simulink model "plantaNeural"  (Simulink 7.4)
settings: Solver=ode45  StartTime=0.0  StopTime=10000  RelTol=1e-3
undefined symbols (not defined in the file or in its folder): now
libraries: neural x29, simulink_extras x2
settings Model: Creator=marco  LastModifiedBy=marco

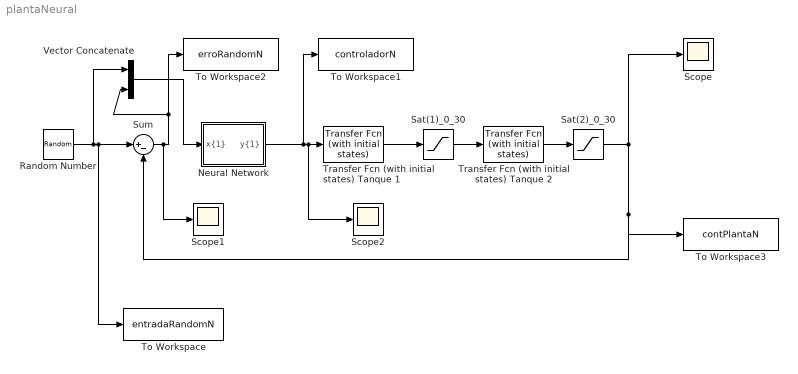
== system plantaNeural ==
  Neural Network : Subsystem
  Random Number : RandomNumber  Mean=15  Variance=15  Seed=round(now)  SampleTime=500
  Sat(1)_0_30 : Saturate  UpperLimit=30  LowerLimit=0  SampleTime=0.1  OutDataType=fixdt(1, 16)  OutScaling=2^0
  Sat(2)_0_30 : Saturate  UpperLimit=30  LowerLimit=0  SampleTime=0.1  OutDataType=fixdt(1, 16)  OutScaling=2^0
  Scope : Scope
  Scope1 : Scope
  Scope2 : Scope
      settings: YMin=4  YMax=5.5  SaveName=ScopeData2
  Sum : Sum  Inputs=|+-  OutDataType=fixdt(1, 16)  OutScaling=2^0  SampleTime=0.1
  To Workspace : ToWorkspace  VariableName=entradaRandomN  SampleTime=0.1  SaveFormat=Array
  To Workspace1 : ToWorkspace  VariableName=controladorN  SampleTime=0.1  SaveFormat=Array
  To Workspace2 : ToWorkspace  VariableName=erroRandomN  SampleTime=0.1  SaveFormat=Array
  To Workspace3 : ToWorkspace  VariableName=contPlantaN  SampleTime=0.1  SaveFormat=Array
  Transfer Fcn (with initial states) Tanque 1 : simulink_extras/Additional Linear/Transfer Fcn (with initial states)  SystemSampleTime=-1  N=[0.2964]  D="[1  0.0656]"  X0=0
  Transfer Fcn (with initial states) Tanque 2 : simulink_extras/Additional Linear/Transfer Fcn (with initial states)  SystemSampleTime=-1  N=[0.0656]  D="[1  0.0656]"  X0=0
  Vector Concatenate : Concatenate  Mode=Vector
  wires:
  Transfer Fcn (with initial states) Tanque 1/1 -> Sat(1)_0_30/1
  Sum/1 -> Scope1/1, To Workspace2/1, Vector Concatenate/2
  Transfer Fcn (with initial states) Tanque 2/1 -> Sat(2)_0_30/1
  Neural Network/1("y{1}") -> To Workspace1/1, Transfer Fcn (with initial states) Tanque 1/1, Scope2/1
  Random Number/1 -> To Workspace/1, Sum/1, Vector Concatenate/1
  Sat(1)_0_30/1 -> Transfer Fcn (with initial states) Tanque 2/1
  Sat(2)_0_30/1 -> Scope/1, Sum/2, To Workspace3/1
  Vector Concatenate/1 -> Neural Network/1("x{1}")

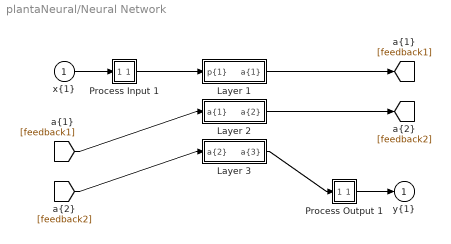
== system plantaNeural/Neural Network ==
  "x{1}" : Inport  PortDimensions=2  SampleTime=1
  Layer 1 : Subsystem
  Layer 2 : Subsystem
  Layer 3 : Subsystem
  Process Input 1 : Subsystem
  Process Output 1 : Subsystem
  "y{1}" : Outport  InitialOutput=0
  wires:
  "x{1}"/1 -> Process Input 1/1(x)
  Process Output 1/1(y) -> "y{1}"/1
  Process Input 1/1(p) -> Layer 1/1("p{1}")
  Layer 1/1("a{1}") -> [feedback1]
  [feedback1] -> Layer 2/1("a{1} ")
  Layer 2/1("a{2}") -> [feedback2]
  [feedback2] -> Layer 3/1("a{2} ")
  Layer 3/1("a{3}") -> Process Output 1/1(a)

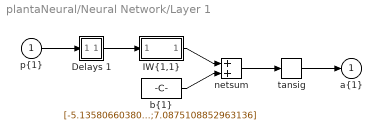
== system plantaNeural/Neural Network/Layer 1 ==
  "p{1}" : Inport  PortDimensions=2  SampleTime=1
  Delays 1 : Subsystem
      mask Display: disp('TDL')
  "IW{1,1}" : Subsystem
      mask Display: disp('weight')
  "b{1}" : Constant  Value=[-5.1358066038064774;-4.3696122158586421;-1.6705858835536853;-2.5464222267076702;-6.160408589801782;0.49822019697729519;-8.1445150751717037;5.2185710150424915;5.2648040348684608;7.0875108852963136]
      mask Display: disp('bias')
  netsum : Sum  Inputs=2  OutDataType=sfix(16)  OutScaling=2^0  SaturateOnIntegerOverflow=on  InputSameDT=on  OutDataTypeStr=Inherit: Same as first input
  tansig : neural/Transfer Functions/tansig  SystemSampleTime=-1
  "a{1}" : Outport  InitialOutput=[0;0;0;0;0;0;0;0;0;0]
  wires:
  "p{1}"/1 -> Delays 1/1("p{1}")
  Delays 1/1("pd{1,1}") -> "IW{1,1}"/1("pd{1,1}")
  "IW{1,1}"/1("iz{1,1}") -> netsum/1
  "b{1}"/1 -> netsum/2
  netsum/1 -> tansig/1
  tansig/1 -> "a{1}"/1

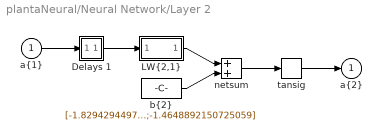
== system plantaNeural/Neural Network/Layer 2 ==
  "a{1} " : Inport  PortDimensions=10  SampleTime=1
  Delays 1 : Subsystem
      mask Display: disp('TDL')
  "LW{2,1}" : Subsystem
      mask Display: disp('weight')
  "b{2}" : Constant  Value=[-1.8294294497199188;2.7561117201367602;-1.1232541464035077;-1.6815661651128024;0.45024471298237856;0.059898257675119207;1.4208618932994941;-4.0307578032176012;0.90781113420925352;-1.4648892150725059]
      mask Display: disp('bias')
  netsum : Sum  Inputs=2  OutDataType=sfix(16)  OutScaling=2^0  SaturateOnIntegerOverflow=on  InputSameDT=on  OutDataTypeStr=Inherit: Same as first input
  tansig : neural/Transfer Functions/tansig  SystemSampleTime=-1
  "a{2}" : Outport  InitialOutput=[0;0;0;0;0;0;0;0;0;0]
  wires:
  "a{1} "/1 -> Delays 1/1("p{2}")
  Delays 1/1("pd{2,1}") -> "LW{2,1}"/1("ad{2,1}")
  "LW{2,1}"/1("lz{2,1}") -> netsum/1
  "b{2}"/1 -> netsum/2
  netsum/1 -> tansig/1
  tansig/1 -> "a{2}"/1

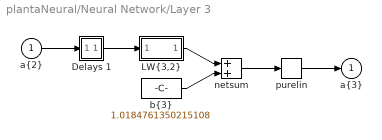
== system plantaNeural/Neural Network/Layer 3 ==
  "a{2} " : Inport  PortDimensions=10  SampleTime=1
  Delays 1 : Subsystem
      mask Display: disp('TDL')
  "LW{3,2}" : Subsystem
      mask Display: disp('weight')
  "b{3}" : Constant  Value=1.0184761350215108
      mask Display: disp('bias')
  netsum : Sum  Inputs=2  OutDataType=sfix(16)  OutScaling=2^0  SaturateOnIntegerOverflow=on  InputSameDT=on  OutDataTypeStr=Inherit: Same as first input
  purelin : neural/Transfer Functions/purelin  SystemSampleTime=-1
  "a{3}" : Outport  InitialOutput=0
  wires:
  "a{2} "/1 -> Delays 1/1("p{3}")
  Delays 1/1("pd{3,2}") -> "LW{3,2}"/1("ad{3,2}")
  "LW{3,2}"/1("lz{3,2}") -> netsum/1
  "b{3}"/1 -> netsum/2
  netsum/1 -> purelin/1
  purelin/1 -> "a{3}"/1

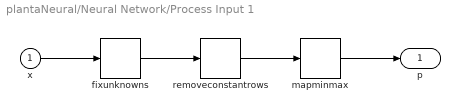
== system plantaNeural/Neural Network/Process Input 1 ==
  x : Inport  PortDimensions=2  SampleTime=1
  fixunknowns : neural/Processing Functions/fixunknowns  SystemSampleTime=-1  dummy=0
  mapminmax : neural/Processing Functions/mapminmax  SystemSampleTime=-1  xmin=[-5.46105933130547;1.67913647989072]  xmax=[23.6732986388822;29.4483698075216]  ymin=-1  ymax=1
  removeconstantrows : neural/Processing Functions/removeconstantrows  SystemSampleTime=-1  inputSize=2  keep=[1 2]
  p : Outport  PortDimensions=2  SampleTime=1
  wires:
  x/1 -> fixunknowns/1
  fixunknowns/1 -> removeconstantrows/1
  removeconstantrows/1 -> mapminmax/1
  mapminmax/1 -> p/1

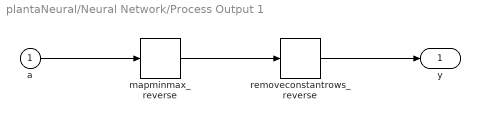
== system plantaNeural/Neural Network/Process Output 1 ==
  a : Inport  PortDimensions=1  SampleTime=1
  mapminmax_reverse : neural/Processing Functions/mapminmax_reverse  SystemSampleTime=-1  xmin=-15  xmax=15  ymin=-1  ymax=1
  removeconstantrows_reverse : neural/Processing Functions/removeconstantrows_reverse  SystemSampleTime=-1  inputSize=1  constants=zeros(0,1)  rearrange=1
  y : Outport  PortDimensions=1  SampleTime=1
  wires:
  a/1 -> mapminmax_reverse/1
  mapminmax_reverse/1 -> removeconstantrows_reverse/1
  removeconstantrows_reverse/1 -> y/1

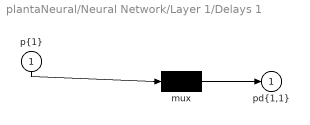
== system plantaNeural/Neural Network/Layer 1/Delays 1 ==
  "p{1}" : Inport  PortDimensions=2  SampleTime=1
  mux : Mux  Inputs=1
  "pd{1,1}" : Outport
  wires:
  "p{1}"/1 -> mux/1
  mux/1 -> "pd{1,1}"/1

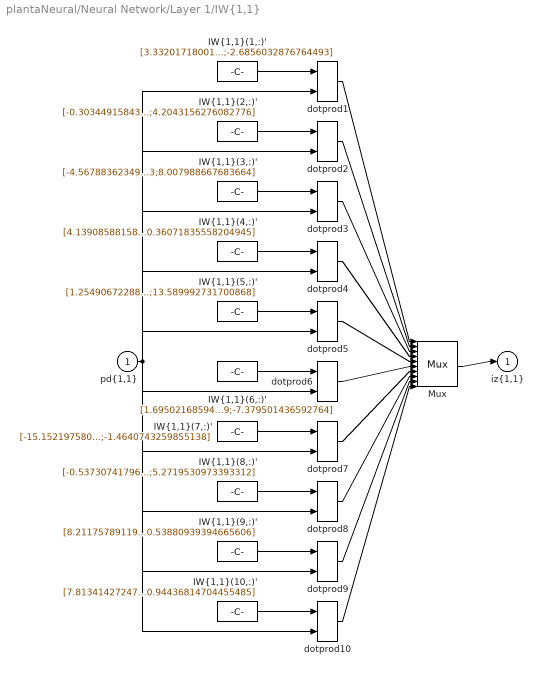
== system plantaNeural/Neural Network/Layer 1/IW{1,1} ==
  "pd{1,1}" : Inport  PortDimensions=2  SampleTime=1
  "IW{1,1}(1,:)'" : Constant  Value=[3.3320171800151712;-2.6856032876764493]
      mask Display: disp('weights')
  "IW{1,1}(10,:)'" : Constant  Value=[7.8134142724702738;0.94436814704455485]
      mask Display: disp('weights')
  "IW{1,1}(2,:)'" : Constant  Value=[-0.3034491584308816;4.2043156276082776]
      mask Display: disp('weights')
  "IW{1,1}(3,:)'" : Constant  Value=[-4.5678836234909763;8.007988667683664]
      mask Display: disp('weights')
  "IW{1,1}(4,:)'" : Constant  Value=[4.139085881580753;-0.36071835558204945]
      mask Display: disp('weights')
  "IW{1,1}(5,:)'" : Constant  Value=[1.2549067228851953;13.589992731700868]
      mask Display: disp('weights')
  "IW{1,1}(6,:)'" : Constant  Value=[1.6950216859409259;-7.379501436592764]
      mask Display: disp('weights')
  "IW{1,1}(7,:)'" : Constant  Value=[-15.152197580993475;-1.4640743259855138]
      mask Display: disp('weights')
  "IW{1,1}(8,:)'" : Constant  Value=[-0.53730741796460768;5.2719530973393312]
      mask Display: disp('weights')
  "IW{1,1}(9,:)'" : Constant  Value=[8.2117578911927342;-0.53880939394665606]
      mask Display: disp('weights')
  Mux : Mux  Inputs=10
  dotprod{1..10} (10 alike) : neural/Weight Functions/dotprod  SystemSampleTime=-1
  "iz{1,1}" : Outport
  wires:
  "IW{1,1}(1,:)'"/1 -> dotprod1/1
  "pd{1,1}"/1 -> dotprod1/2, dotprod2/2, dotprod3/2, dotprod4/2, dotprod5/2, dotprod6/2, dotprod7/2, dotprod8/2, dotprod9/2, dotprod10/2
  dotprod1/1 -> Mux/1
  "IW{1,1}(2,:)'"/1 -> dotprod2/1
  dotprod2/1 -> Mux/2
  "IW{1,1}(3,:)'"/1 -> dotprod3/1
  dotprod3/1 -> Mux/3
  "IW{1,1}(4,:)'"/1 -> dotprod4/1
  dotprod4/1 -> Mux/4
  "IW{1,1}(5,:)'"/1 -> dotprod5/1
  dotprod5/1 -> Mux/5
  "IW{1,1}(6,:)'"/1 -> dotprod6/1
  dotprod6/1 -> Mux/6
  "IW{1,1}(7,:)'"/1 -> dotprod7/1
  dotprod7/1 -> Mux/7
  "IW{1,1}(8,:)'"/1 -> dotprod8/1
  dotprod8/1 -> Mux/8
  "IW{1,1}(9,:)'"/1 -> dotprod9/1
  dotprod9/1 -> Mux/9
  "IW{1,1}(10,:)'"/1 -> dotprod10/1
  dotprod10/1 -> Mux/10
  Mux/1 -> "iz{1,1}"/1

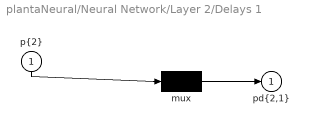
== system plantaNeural/Neural Network/Layer 2/Delays 1 ==
  "p{2}" : Inport  PortDimensions=10  SampleTime=1
  mux : Mux  Inputs=1
  "pd{2,1}" : Outport
  wires:
  "p{2}"/1 -> mux/1
  mux/1 -> "pd{2,1}"/1

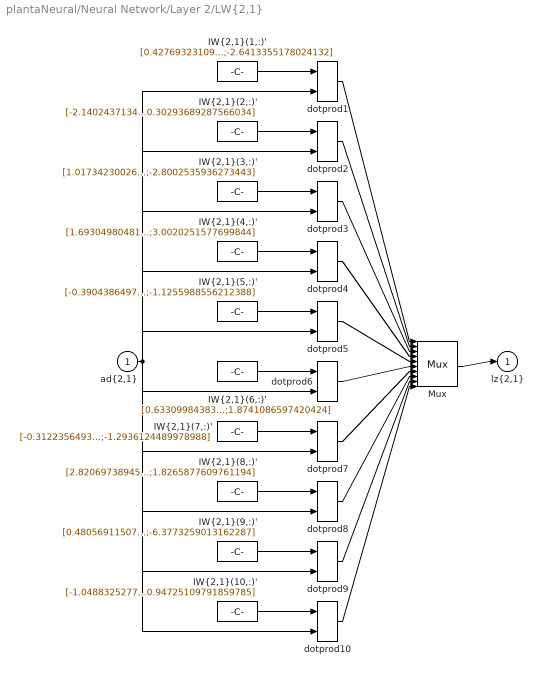
== system plantaNeural/Neural Network/Layer 2/LW{2,1} ==
  "ad{2,1}" : Inport  PortDimensions=10  SampleTime=1
  "IW{2,1}(1,:)'" : Constant  Value=[0.42769323109441454;1.0677518796008716;-9.678408334989328;-0.44202834872680907;-2.2384900678786295;2.2189493171745078;7.6109778678760796;-1.4765313790733037;-16.48331783614772;-2.6413355178024132]
      mask Display: disp('weights')
  "IW{2,1}(10,:)'" : Constant  Value=[-1.0488325277005255;-3.41501801059206;1.3545111177456501;-0.39876233888838603;-4.5607611860595334;1.4536504569648081;3.8170953556686729;0.96206896487905424;0.7007939194977979;0.94725109791859785]
      mask Display: disp('weights')
  "IW{2,1}(2,:)'" : Constant  Value=[-2.1402437134918113;-0.56447953546496432;0.36697284940864405;-1.2422781143811115;-1.6135934144662236;3.8897412846254769;0.15219906792044915;0.25239920019752793;4.1257670120331031;0.30293689287566034]
      mask Display: disp('weights')
  "IW{2,1}(3,:)'" : Constant  Value=[1.0173423002617004;-1.0377455351706311;3.2305855154907448;0.54004854868273477;1.6759705714495812;4.6832376313882484;3.4306837122802856;0.95007526481674343;0.96354376225145066;-2.8002535936273443]
      mask Display: disp('weights')
  "IW{2,1}(4,:)'" : Constant  Value=[1.6930498048100069;-1.9985423706215186;-2.7334269849726156;0.65528073194466185;-4.0416192207881441;-7.9474198410198253;-3.2038989277157763;0.88629071098925594;1.1131350347955884;3.0020251577699844]
      mask Display: disp('weights')
  "IW{2,1}(5,:)'" : Constant  Value=[-0.39043864979938769;-6.0592870126288103;0.30624934298739659;-1.3365257291757009;-4.7957891383078781;0.89552112298869291;3.3047084999455478;-0.92512347656969462;-0.10272630958694136;-1.1255988556212388]
      mask Display: disp('weights')
  "IW{2,1}(6,:)'" : Constant  Value=[0.63309984383899698;-0.52819234631307665;0.71605883786708835;0.28858604770856794;0.48104136151786753;2.2308019679502675;-2.5919219963543823;1.0368380167106572;0.84802963849658319;1.8741086597420424]
      mask Display: disp('weights')
  "IW{2,1}(7,:)'" : Constant  Value=[-0.3122356493616178;1.9523767854449963;-1.3898653528183145;-0.30522483561694791;-0.44457503776175183;-2.5183928744685513;2.3657005887251286;-0.91057543136421493;-0.93615495580077579;-1.2936124489978988]
      mask Display: disp('weights')
  "IW{2,1}(8,:)'" : Constant  Value=[2.820697389454498;-4.7959251280705981;6.9083660064056529e-007;2.3113698574500727;0.46687273804800056;0.096609540379576933;3.4265637548804531;-2.3783144493583426;-2.0547233803194764;1.8265877609761194]
      mask Display: disp('weights')
  "IW{2,1}(9,:)'" : Constant  Value=[0.48056911507037509;1.4718585987861426;5.4871310552901207;0.66812728449489645;-0.42533311983851985;10.594028795666221;3.0366133282205787;0.22673875459482323;0.69517063427310655;-6.3773259013162287]
      mask Display: disp('weights')
  Mux : Mux  Inputs=10
  dotprod{1..10} (10 alike) : neural/Weight Functions/dotprod  SystemSampleTime=-1
  "lz{2,1}" : Outport
  wires:
  "IW{2,1}(1,:)'"/1 -> dotprod1/1
  "ad{2,1}"/1 -> dotprod1/2, dotprod2/2, dotprod3/2, dotprod4/2, dotprod5/2, dotprod6/2, dotprod7/2, dotprod8/2, dotprod9/2, dotprod10/2
  dotprod1/1 -> Mux/1
  "IW{2,1}(2,:)'"/1 -> dotprod2/1
  dotprod2/1 -> Mux/2
  "IW{2,1}(3,:)'"/1 -> dotprod3/1
  dotprod3/1 -> Mux/3
  "IW{2,1}(4,:)'"/1 -> dotprod4/1
  dotprod4/1 -> Mux/4
  "IW{2,1}(5,:)'"/1 -> dotprod5/1
  dotprod5/1 -> Mux/5
  "IW{2,1}(6,:)'"/1 -> dotprod6/1
  dotprod6/1 -> Mux/6
  "IW{2,1}(7,:)'"/1 -> dotprod7/1
  dotprod7/1 -> Mux/7
  "IW{2,1}(8,:)'"/1 -> dotprod8/1
  dotprod8/1 -> Mux/8
  "IW{2,1}(9,:)'"/1 -> dotprod9/1
  dotprod9/1 -> Mux/9
  "IW{2,1}(10,:)'"/1 -> dotprod10/1
  dotprod10/1 -> Mux/10
  Mux/1 -> "lz{2,1}"/1

== system plantaNeural/Neural Network/Layer 3/Delays 1 ==
  "p{3}" : Inport  PortDimensions=10  SampleTime=1
  mux : Mux  Inputs=1
  "pd{3,2}" : Outport
  wires:
  "p{3}"/1 -> mux/1
  mux/1 -> "pd{3,2}"/1

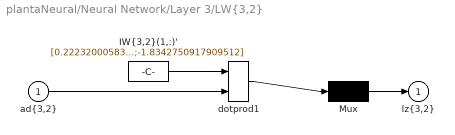
== system plantaNeural/Neural Network/Layer 3/LW{3,2} ==
  "ad{3,2}" : Inport  PortDimensions=10  SampleTime=1
  "IW{3,2}(1,:)'" : Constant  Value=[0.22232000583033265;-4.9441005154036626;-1.99857846481166;3.507350841906423;1.8279860158278314;-3.2821977292483799;-3.7264106289282664;-3.9351121671962614;4.728430137709247;-1.8342750917909512]
      mask Display: disp('weights')
  Mux : Mux  Inputs=1
  dotprod1 : neural/Weight Functions/dotprod  SystemSampleTime=-1
  "lz{3,2}" : Outport
  wires:
  "IW{3,2}(1,:)'"/1 -> dotprod1/1
  "ad{3,2}"/1 -> dotprod1/2
  dotprod1/1 -> Mux/1
  Mux/1 -> "lz{3,2}"/1
